simulink model "modelo_f_HIL_ST"  (R2024b)
settings: Solver=ode15s  StartTime=0.0  StopTime=inf  FixedStep=T_s  RelTol=1e-3
InitFcn:
  | clc
  | clear
  | close all
  | clear all
  | clear mex
  | parametros
  | gain_CL
  | calculo_observador_carro
  | calculo_observador_izaje
values from neighbouring files (symbols this model uses):
  b_cx = 1e6    (= 1000000)    [parametros.m]
  b_cy = 1e7    (= 10000000)    [parametros.m]
  b_hb = 1e8    (= 100000000)    [parametros.m]
  b_hd = 8    [parametros.m]
  b_hm = 18    [parametros.m]
  b_t = 90    [parametros.m]
  b_tb = 5e6    (= 5000000)    [parametros.m]
  b_td = 1.8    [parametros.m]
  b_tm = 6    [parametros.m]
  b_tw = 3e3    (= 3000)    [parametros.m]
  b_wu = 150    [parametros.m]
  container_pillars = container_pillars(randperm(19))    [parametros.m]
  escenario = 1    [parametros.m]
  g = 9.80665    [parametros.m]
  H_c = 2.59    [parametros.m]
  H_truck = 1    [parametros.m]
  i_h = 22    [parametros.m]
  i_t = 30    [parametros.m]
  J_hd_hEb = 3800    [parametros.m]
  J_hm_hb = 30    [parametros.m]
  J_td = 1200    [parametros.m]
  J_tm_tb = 7    [parametros.m]
  K_cy = 1.8e9    (= 1800000000)    [parametros.m]
  K_tw = 4.8e5    (= 480000)    [parametros.m]
  k_wu = 2.36e8    (= 236000000)    [parametros.m]
  l_h0 = (Y_t0-y_l0)    (= 38)    [parametros.m]
  l_h_max = Y_t0-y_h_min    (= 65)    [parametros.m]
  l_h_maxE = l_h_max+0.5    (= 65.5)    [parametros.m]
  l_h_min = Y_t0-y_h_max    (= 5)    [parametros.m]
  l_h_minE = l_h_min-0.5    (= 4.5)    [parametros.m]
  M_cmax = 50000    [parametros.m]
  M_cmin = 2000    [parametros.m]
  M_s = 15000    [parametros.m]
  M_t = 30000    [parametros.m]
  r_hd = 0.75    [parametros.m]
  r_td = 0.50    (= 0.5)    [parametros.m]
  T_hbMax = 5e4    (= 50000)    [parametros.m]
  T_hEbMax = 1.1e6    (= 1100000)    [parametros.m]
  T_hmMax = 2e4    (= 20000)    [parametros.m]
  T_s = 0.001    [parametros.m]
  T_s0 = 0.001    [parametros.m]
  T_s1 = 0.020    (= 0.02)    [parametros.m]
  T_s2 = 0.020    (= 0.02)    [parametros.m]
  T_tbMax = 5e3    (= 5000)    [parametros.m]
  T_tmMax = 4e3    (= 4000)    [parametros.m]
  tau_tm = 1e-3    (= 0.001)    [parametros.m]
  theta_hm0 = -l_h0*i_h*2/r_hd    (= -2229.33333333)    [parametros.m]
  theta_tm0 = (x_t0)*i_t/r_td    (= -900)    [parametros.m]
  trucks0 = [0, 0, 0, 0, 0]    [parametros.m]
  v_h_max_load = 1.5    [parametros.m]
  v_h_max_noload = 3    [parametros.m]
  v_lx0 = 0    [parametros.m]
  v_ly0 = 0    [parametros.m]
  v_t0 = 0    [parametros.m]
  v_t_max = 4    [parametros.m]
  W_c = ctrb(A, B_c(:,1))    [CyO_carro.m]    (also in CyO_izaje.m; parametros.m = 2.44)
  w_hm0 = 0    [parametros.m]
  w_hm_rated = v_h_max_load*2*i_h/r_hd    (= 88)    [parametros.m]
  w_tm0 = (v_t0)*i_t/r_td    (= 0)    [parametros.m]
  x_c0_left = -35    [parametros.m]
  x_c0_right = 55    [parametros.m]
  x_containers_left_lim = 1.5    [parametros.m]
  x_containers_right_lim = 48.5    [parametros.m]
  x_l0 = x_t0    (= -15)    [parametros.m]
  x_lidar_offset = 3.0    (= 3)    [parametros.m]
  x_t0 = -15    [parametros.m]
  x_t_max = 50    [parametros.m]
  x_t_maxE = x_t_max+0.5    (= 50.5)    [parametros.m]
  x_t_min = -30    [parametros.m]
  x_t_minE = x_t_min-0.5    (= -30.5)    [parametros.m]
  y_h_min = -20    [parametros.m]
  y_l0 = 7    [parametros.m]
  Y_sb = 5.0    (= 5)    [parametros.m]
  Y_t0 = 45    [parametros.m]
libraries: opcualib x2, dspnetwork x2, dspsigops x1, simulink x1
(part 2 of 3)

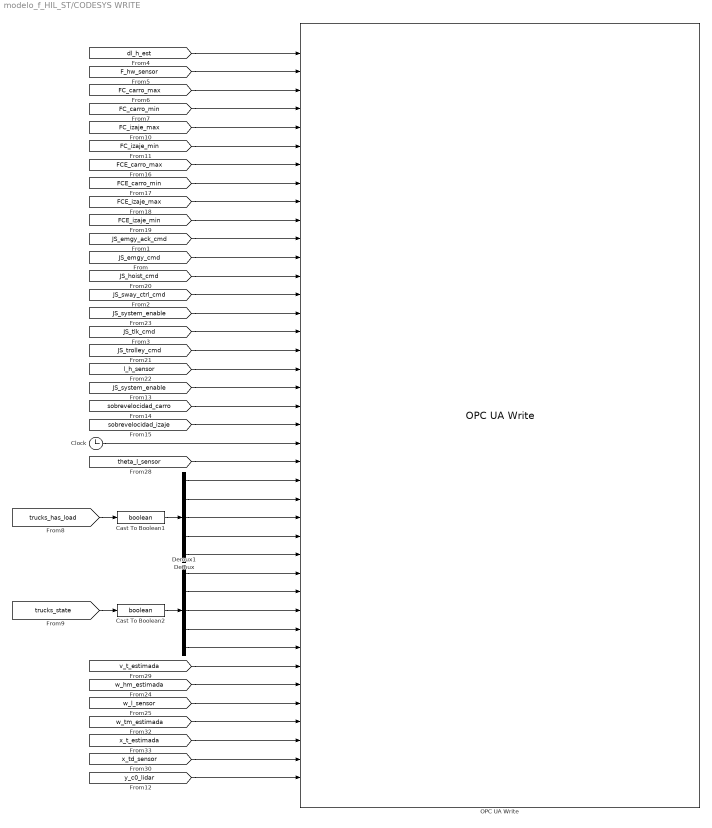
== system modelo_f_HIL_ST/CODESYS WRITE ==
  Cast To Boolean1 : DataTypeConversion  OutDataTypeStr=boolean  SaturateOnIntegerOverflow=off  RndMeth=Floor
  Cast To Boolean2 : DataTypeConversion  OutDataTypeStr=boolean  SaturateOnIntegerOverflow=off  RndMeth=Floor
  Clock : Clock
      settings: Decimation=1/T_s1
  Demux : Demux  Outputs=5
  Demux1 : Demux  Outputs=5
  OPC UA Write : opcualib/OPC UA Write  SelectedServer=OPCUAServer@DESKTOP-IGNACIOMARTINDUCI  ServerList=OPCUAServer@DESKTOP-IGNACIOMARTINDUCI  SampleTime=T_s1  NodeList={ '1', 'dl_h_est', '4', '|var|CODESYS Control Win V3 x64.Application_ST.GVL_VARS.dl_h_est', '0'; '2', 'F_hw_sensor', '4', '|var|CODESYS Control Win V3 x64.Application_ST.GVL_VARS.F_hw_sensor', '0'; '3', 'FC_carro_max', '4', '|var|CODESYS Control Win V3 x64.Application_ST.GVL_VARS.FC_carro_max', '0'; '4', 'FC_carro_min', '4', '|var|CODESYS Control Win V3 x64.Application_ST.GVL_VARS.FC_carro_min', '0'; '5', 'FC_izaje_max', '4', '|var|CODESYS Control Win V3 x64.Application_ST.GVL_VARS.FC_izaje_max', '0'; '6', 'FC_izaje_min', '4', '|var|CODESYS Control Win V3 x64.Application_ST.GVL_VARS.FC_izaje_min', '0'; '7', 'FCE_carro_max', '4', '|var|CODESYS Control Win V3 x64.Application_ST.GVL_VARS.FCE_carro_max', '0'; '8', 'FCE_carro_min', '4', '|var|CODESYS Control Win V3 x64.Application_ST.GVL_VARS.FCE_carro_min', '0'; '9', 'FCE_izaje_max', '4', '|var|CODESYS Control Win V3 x64.Application_ST.GVL_VARS.FCE_izaje_max', '0'; '10', 'FCE_izaje_min', '4', '|var|CODESYS Control Win V3 x64.Application_ST.GVL_VARS.FCE_izaje_min', '0'; '11', 'JS_emgy_ack_cmd', '4', '|var|CODESYS Control Win V3 x64.Application_ST.GVL_VARS.JS_emgy_ack_cmd', '0'; '12', 'JS_emgy_cmd', '4', '|var|CODESYS Control Win V3 x64.Application_ST.GVL_VARS.JS_emgy_cmd', '0'; '13', 'JS_hoist_cmd', '4', '|var|CODESYS Control Win V3 x64.Application_ST.GVL_VARS.JS_hoist_cmd', '0'; '14', 'JS_sway_ctrl_cmd', '4', '|var|CODESYS Control Win V3 x64.Application_ST.GVL_VARS.JS_sway_ctrl_cmd', '0'; '15', 'JS_system_enable', '4', '|var|CODESYS Control Win V3 x64.Application_ST.GVL_VARS.JS_system_enable', '0'; '16', 'JS_tlk_cmd', '4', '|var|CODESYS Control Win V3 x64.Application_ST.GVL_VARS.JS_tlk_cmd', '0'; '17', 'JS_trolley_cmd', '4', '|var|CODESYS Control Win V3 x64.Application_ST.GVL_VARS.JS_trolley_cmd', '0'; '18', 'l_h_sensor', '4', '|var|CODESYS Control Win V3 x64.Application_ST.GVL_VARS.l_h_sensor', '0'; '19', 'P_APN', '4', '|var|CODESYS Control Win V3 x64.Application_ST.GVL_VARS.P_APN', '0'; '20', 'sobrevelocidad_carro', '4', '|var|CODESYS Control Win V3 x64.Application_ST.GVL_VARS.sobrevelocidad_carro', '0'; '21', 'sobrevelocidad_izaje', '4', '|var|CODESYS Control Win V3 x64.Application_ST.GVL_VARS.sobrevelocidad_izaje', '0'; '22', 't', '4', '|var|CODESYS Control Win V3 x64.Application_ST.GVL_VARS.t', '0'; '23', 'theta_l_sensor', '4', '|var|CODESYS Control Win V3 x64.Application_ST.GVL_VARS.theta_l_sensor', '0'; '24', 'THL_1', '4', '|var|CODESYS Control Win V3 x64.Application_ST.GVL_VARS.THL_1', '0'; '25', 'THL_2', '4', '|var|CODESYS Control Win V3 x64.Application_ST.GVL_VARS.THL_2', '0'; '26', 'THL_3', '4', '|var|CODESYS Control Win V3 x64.Application_ST.GVL_VARS.THL_3', '0'; '27', 'THL_4', '4', '|var|CODESYS Control Win V3 x64.Application_ST.GVL_VARS.THL_4', '0'; '28', 'THL_5', '4', '|var|CODESYS Control Win V3 x64.Application_ST.GVL_VARS.THL_5', '0'; '29', 'TS_1', '4', '|var|CODESYS Control Win V3 x64.Application_ST.GVL_VARS.TS_1', '0'; '30', 'TS_2', '4', '|var|CODESYS Control Win V3 x64.Application_ST.GVL_VARS.TS_2', '0'; '31', 'TS_3', '4', '|var|CODESYS Control Win V3 x64.Application_ST.GVL_VARS.TS_3', '0'; '32', 'TS_4', '4', '|var|CODESYS Control Win V3 x64.Application_ST.GVL_VARS.TS_4', '0'; '33', 'TS_5', '4', '|var|CODESYS Control Win V3 x64.Application_ST.GVL_VARS.TS_5', '0'; '34', 'v_t_est', '4', '|var|CODESYS Control Win V3 x64.Application_ST.GVL_VARS.v_t_est', '0'; '35', 'w_hm_estimada', '4', '|var|CODESYS Control Win V3 x64.Application_ST.GVL_VARS.w_hm_estimada', '0'; '36', 'w_l_sensor', '4', '|var|CODESYS Control Win V3 x64.Application_ST.GVL_VARS.w_l_sensor', '0'; '37', 'w_tm_estimada', '4', '|var|CODESYS Control Win V3 x64.Application_ST.GVL_VARS.w_tm_estimada', '0'; '38', 'x_t_est', '4', '|var|CODESYS Control Win V3 x64.Application_ST.GVL_VARS.x_t_est', '0'; '39', 'x_td_sensor', '4', '|var|CODESYS Control Win V3 x64.Application_ST.GVL_VARS.x_td_sensor', '0'; '40', 'y_c0_lidar', '4', '|var|CODESYS Control Win V3 x64.Application_ST.GVL_VARS.y_c0_lidar', '0' }
  wires:
  [dl_h_est] -> OPC UA Write/1
  [F_hw_sensor] -> OPC UA Write/2
  [trucks_has_load] -> Cast To Boolean1/1
  Cast To Boolean1/1 -> Demux/1
  [trucks_state] -> Cast To Boolean2/1
  Cast To Boolean2/1 -> Demux1/1
  [FC_carro_max] -> OPC UA Write/3
  [FC_carro_min] -> OPC UA Write/4
  [FC_izaje_min] -> OPC UA Write/6
  [FCE_carro_min] -> OPC UA Write/8
  [FC_izaje_max] -> OPC UA Write/5
  [FCE_izaje_max] -> OPC UA Write/9
  [FCE_carro_max] -> OPC UA Write/7
  [FCE_izaje_min] -> OPC UA Write/10
  [JS_emgy_ack_cmd] -> OPC UA Write/11
  [JS_emgy_cmd] -> OPC UA Write/12
  [JS_hoist_cmd] -> OPC UA Write/13
  [JS_sway_ctrl_cmd] -> OPC UA Write/14
  [JS_system_enable] -> OPC UA Write/15
  [JS_tlk_cmd] -> OPC UA Write/16
  [JS_trolley_cmd] -> OPC UA Write/17
  [l_h_sensor] -> OPC UA Write/18
  [JS_system_enable] -> OPC UA Write/19
  [sobrevelocidad_carro] -> OPC UA Write/20
  [sobrevelocidad_izaje] -> OPC UA Write/21
  Clock/1 -> OPC UA Write/22
  [theta_l_sensor] -> OPC UA Write/23
  [v_t_estimada] -> OPC UA Write/34
  [w_hm_estimada] -> OPC UA Write/35
  [w_l_sensor] -> OPC UA Write/36
  [w_tm_estimada] -> OPC UA Write/37
  [x_t_estimada] -> OPC UA Write/38
  [x_td_sensor] -> OPC UA Write/39
  [y_c0_lidar] -> OPC UA Write/40
  Demux/1 -> OPC UA Write/24
  Demux/2 -> OPC UA Write/25
  Demux/3 -> OPC UA Write/26
  Demux/4 -> OPC UA Write/27
  Demux/5 -> OPC UA Write/28
  Demux1/1 -> OPC UA Write/29
  Demux1/2 -> OPC UA Write/30
  Demux1/3 -> OPC UA Write/31
  Demux1/4 -> OPC UA Write/32
  Demux1/5 -> OPC UA Write/33

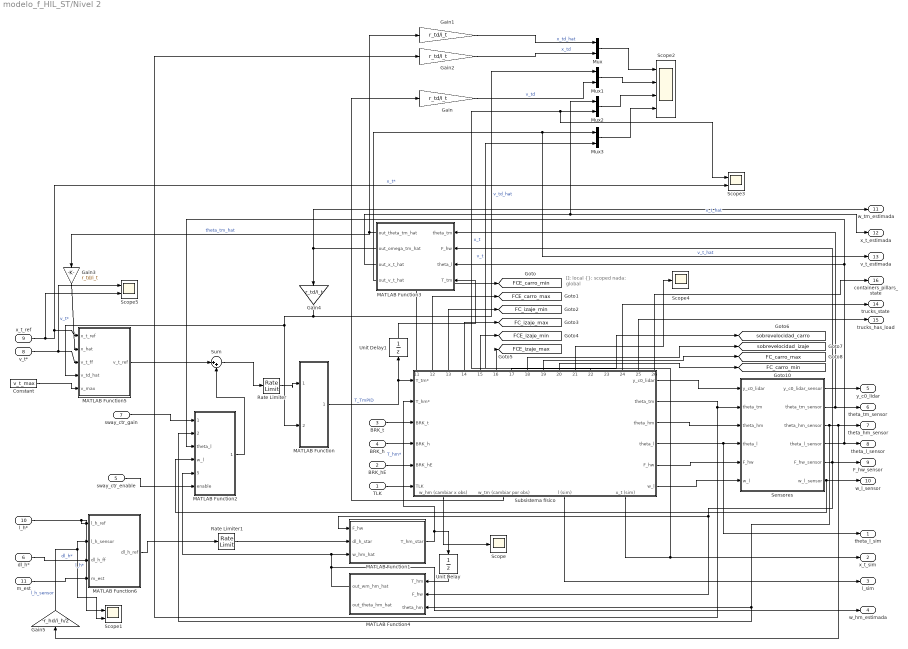
== system modelo_f_HIL_ST/Nivel 2 ==
  note: []: local
      | {}: scoped
      | nada: global
  TLK : Inport
  BRK_hE : Inport  Port=2
  BRK_t : Inport  Port=3
  BRK_h : Inport  Port=4
  sway_ctr_enable : Inport  Port=5
  dl_h* : Inport  Port=6
  sway_ctr_gain : Inport  Port=7
  v_t* : Inport  Port=8
  x_t_ref : Inport  Port=9
  l_h* : Inport  Port=10
  m_est : Inport  Port=11
  Constant : Constant  Value=v_t_max
  Gain{,1..4} (5 alike) : Gain  Gain=r_td/i_t
  Gain5 : Gain  Gain=-r_hd/i_h/2
  MATLAB Function : MATLAB Function  TreatAsAtomicUnit=on  SystemSampleTime=T_s0
  MATLAB Function1 : MATLAB Function  TreatAsAtomicUnit=on  SystemSampleTime=T_s0
  MATLAB Function2 : MATLAB Function  TreatAsAtomicUnit=on  SystemSampleTime=T_s0
  MATLAB Function3 : MATLAB Function  TreatAsAtomicUnit=on  SystemSampleTime=T_s0
  MATLAB Function4 : MATLAB Function  TreatAsAtomicUnit=on  SystemSampleTime=T_s0
  MATLAB Function5 : MATLAB Function  TreatAsAtomicUnit=on
  MATLAB Function6 : MATLAB Function  TreatAsAtomicUnit=on
  Mux{,1..3} (4 alike) : Mux  Inputs=2
  Rate Limiter : RateLimiter  RisingSlewLimit=0.8  FallingSlewLimit=-0.8  SampleTimeMode=inherited  InitialCondition=T_s
  Rate Limiter1 : RateLimiter  RisingSlewLimit=0.75  FallingSlewLimit=-0.75  SampleTimeMode=inherited  InitialCondition=T_s
  Scope : Scope
  Scope1 : Scope  NumInputPorts=2
  Scope2 : Scope  NumInputPorts=4
  Scope3 : Scope  NumInputPorts=2
  Scope4 : Scope
  Scope5 : Scope  NumInputPorts=2
  Sensores : Subsystem
  Subsistema físico : Subsystem
      settings: PortSchema="{\"entries\":[{\"content\":{\"sides\":[{\"content\":{\"connectorIds\":[\"In1\",\"In2\",\"In3\",\"In4\",\"In5\",\"In6\"]},\"type\":\"ConnectorPlacement.EquallySpacedRectSide\",\"uuid\":\"aa1cb789-2051-45a4-8cb8-6dd2078290cc\"},{\"content\":{\"connectorIds\":[\"Out1\",\"Out2\",\"Out3\",\"Out4\",\"Out5\",\"Out6\"],\"side\":\"RIGHT\"},\"type\":\"ConnectorPlacement.EquallySpacedRectSide\",\"uuid\":\"7fe62279-dd3b-46db-ba9e-e4633dcea5c6\"},{\"content\":{\"connectorIds\":[\"Out11\",\"Out12\",\"Out13\",\"Out14\",\"Out15\",\"Out16\",\"Out17\",\"Out18\",\"Out19\",\"Out20\",\"Out21\",\"Out22\",\"Out23\",\"Out24\",\"Out25\",\"Out26\"],\"side\":\"TOP\"},\"type\":\"ConnectorPlacement.EquallySpacedRectSide\",\"uuid\":\"a5663ea7-10d8-47d7-b8ed-8fbfb239b85a\"},{\"content\":{\"connectorIds\":[\"Out7\",\"Out8\",\"Out9\",\"Out10\"],\"side\":\"BOTTOM\"},\"type\":\"ConnectorPlacement.EquallySpacedRectSide\",\"uuid\":\"9ec9131f-7b2f-42d7-8a86-9462c3c282b3\"}]},\"type\":\"ConnectorPlacement.EquallySpacedConnector\",\"uuid\":\"e7df1a56-7803-4e0d-8bf9-081877eb8c08\"}],\"packageUris\":[\"http://schema.mathworks.com/mf0/Connector/R2020b\"],\"version\":\"1.0\"}"
  Sum : Sum  Inputs=|++
  Unit Delay : UnitDelay  SampleTime=T_s  HasFrameUpgradeWarning=on
  Unit Delay1 : UnitDelay  SampleTime=T_s  HasFrameUpgradeWarning=on
  theta_l_sim : Outport
  x_t_sim : Outport  Port=2
  l_sim : Outport  Port=3
  w_hm_estimada : Outport  Port=4
  y_c0_lidar : Outport  Port=5
  theta_tm_sensor : Outport  Port=6
  theta_hm_sensor : Outport  Port=7
  theta_l_sensor : Outport  Port=8
  F_hw_sensor : Outport  Port=9
  w_l_sensor : Outport  Port=10
  w_tm_estimada : Outport  Port=11
  x_t_estimada : Outport  Port=12
  v_t_estimada : Outport  Port=13
  trucks_state : Outport  Port=14
  trucks_has_load : Outport  Port=15
  containers_pillars_state : Outport  Port=16
  tag scope: FCE_carro_max=global, FCE_carro_min=global, FCE_izaje_max=global, FCE_izaje_min=global, FC_carro_max=global, FC_carro_min=global, FC_izaje_max=global, FC_izaje_min=global, sobrevelocidad_carro=global, sobrevelocidad_izaje=global
  wires:
  Sensores/5(F_hw_sensor) -> F_hw_sensor/1, MATLAB Function4/2(F_hw), MATLAB Function1/1(F_hw), MATLAB Function3/2(F_hw)
  Sensores/2(theta_tm_sensor) -> theta_tm_sensor/1, MATLAB Function3/1(theta_tm)
  Subsistema físico/19(FC_carro_max) -> [FC_carro_max]
  Sensores/3(theta_hm_sensor) -> theta_hm_sensor/1, Gain5/1, MATLAB Function4/3(theta_hm), MATLAB Function2/2(theta_hm)
  Sensores/6(w_l_sensor) -> w_l_sensor/1, MATLAB Function2/4(w_l)
  Subsistema físico/15(FCE_izaje_min) -> [FCE_izaje_min]
  Unit Delay/1 -> MATLAB Function4/1(T_hm)
  Subsistema físico/13(FC_izaje_min) -> [FC_izaje_min]
  Subsistema físico/16(FCE_izaje_max) -> [FCE_izaje_max]
  MATLAB Function1/1(T_hm_star) -> Unit Delay/1, Subsistema físico/2(T_hm*)  "T_hm*"
  Subsistema físico/6(w_l) -> Sensores/6(w_l)
  Subsistema físico/17(sobrevelocidad_carro) -> [sobrevelocidad_carro]
  Subsistema físico/3(theta_hm) -> Sensores/3(theta_hm)
  MATLAB Function4/1(out_wm_hm_hat) -> MATLAB Function2/5(w_hm_hat), MATLAB Function1/3(w_hm_hat), w_hm_estimada/1
  dl_h*/1 -> MATLAB Function6/3(dl_h_ff)  "dl_h*"
  Subsistema físico/1(y_c0_lidar) -> Sensores/1(y_c0_lidar)
  Subsistema físico/5(F_hw) -> Sensores/5(F_hw)
  Subsistema físico/2(theta_tm) -> Gain2/1, Sensores/2(theta_tm)
  Subsistema físico/18(sobrevelocidad_izaje) -> [sobrevelocidad_izaje]
  Subsistema físico/11(FCE_carro_min) -> [FCE_carro_min]
  Subsistema físico/4(theta_l) -> theta_l_sim/1, Sensores/4(theta_l)
  Subsistema físico/14(FC_izaje_max) -> [FC_izaje_max]
  Subsistema físico/20(FC_carro_min) -> [FC_carro_min]
  Subsistema físico/12(FCE_carro_max) -> [FCE_carro_max]
  BRK_t/1 -> Subsistema físico/3(BRK_t)
  BRK_h/1 -> Subsistema físico/4(BRK_h)
  BRK_hE/1 -> Subsistema físico/5(BRK_hE)
  TLK/1 -> Subsistema físico/6(TLK)
  Sensores/1(y_c0_lidar_sensor) -> y_c0_lidar/1
  sway_ctr_enable/1 -> MATLAB Function2/6(enable)
  MATLAB Function3/2(out_omega_tm_hat) -> w_tm_estimada/1, Gain4/1
  Gain4/1 -> Mux1/1, MATLAB Function5/4(v_td_hat), MATLAB Function/2(v_td_hat)  "v_td_hat"
  MATLAB Function5/1(v_t_ref) -> Sum/1
  Sensores/4(theta_l_sensor) -> theta_l_sensor/1, MATLAB Function2/3(theta_l), MATLAB Function3/3(theta_l)
  Unit Delay1/1 -> MATLAB Function3/4(T_tm)
  Subsistema físico/10(x_t (sim)) -> Scope3/1, Mux2/2, x_t_sim/1  "x_t"
  Subsistema físico/9(l (sim)) -> l_sim/1
  MATLAB Function3/3(out_x_t_hat) -> x_t_estimada/1, Mux2/1  "x_t_hat"
  Subsistema físico/22(v_t (sim)) -> Mux3/2  "v_t"
  Subsistema físico/8(w_tm (cambiar por obs)) -> Gain/1
  Gain/1 -> Mux1/2  "v_td"
  MATLAB Function3/1(out_theta_tm_hat) -> Gain3/1, Gain1/1  "theta_tm_hat"
  Gain1/1 -> Mux/1  "x_td_hat"
  Gain2/1 -> Mux/2  "x_td"
  MATLAB Function3/4(out_v_t_hat) -> v_t_estimada/1, Mux3/1  "v_t_hat"
  Mux/1 -> Scope2/1
  Mux1/1 -> Scope2/2
  Mux3/1 -> Scope2/4
  Mux2/1 -> Scope2/3
  Subsistema físico/24(trucks_state) -> trucks_state/1
  x_t_ref/1 -> Scope5/2, Scope3/2, MATLAB Function5/1(x_t_ref)  "x_t*"
  sway_ctr_gain/1 -> MATLAB Function2/1(sway_ctr_gain)
  Subsistema físico/25(trucks_has_load) -> trucks_has_load/1
  MATLAB Function/1(T_tm_star) -> Unit Delay1/1, Subsistema físico/1(T_tm*)  "T_TmPID"
  MATLAB Function2/1(v_balanceo) -> Sum/2
  Sum/1 -> Rate Limiter/1
  v_t*/1 -> Scope5/1, MATLAB Function5/3(v_t_ff)  "v_t*"
  Constant/1 -> MATLAB Function5/5(v_max)
  Gain3/1 -> MATLAB Function5/2(x_hat)
  Subsistema físico/7(w_hm (cambiar x obs)) -> Scope/1
  Gain5/1 -> Scope1/2, MATLAB Function6/2(l_h_sensor)  "l_h_sensor"
  l_h*/1 -> Scope1/1, MATLAB Function6/1(l_h_ref)  "l_h*"
  MATLAB Function6/1(dl_h_ref) -> Rate Limiter1/1
  Rate Limiter/1 -> MATLAB Function/1(v_t_star)
  Rate Limiter1/1 -> MATLAB Function1/2(dl_h_star)
  Subsistema físico/26(containers_pillars_state) -> containers_pillars_state/1
  Subsistema físico/21(m_l (sim)) -> Scope4/1
  m_est/1 -> MATLAB Function6/4(m_est)

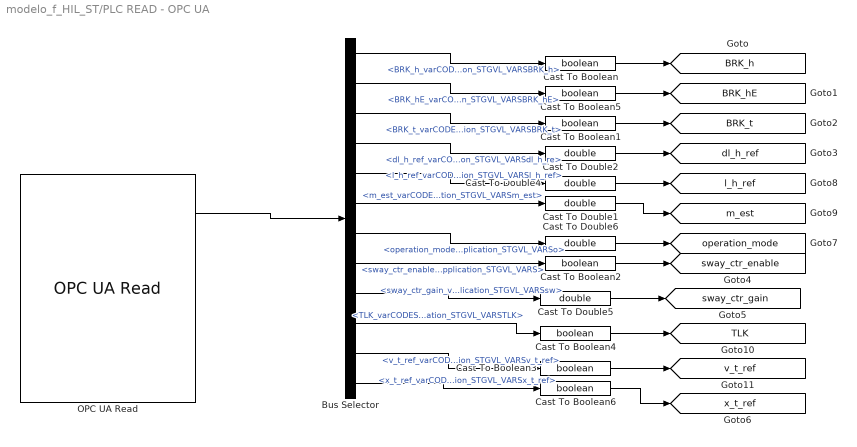
== system modelo_f_HIL_ST/PLC READ - OPC UA ==
  Bus Selector : BusSelector  OutputSignals=BRK_h_varCODESYSControlWinV3X64Application_STGVL_VARSBRK_h,BRK_hE_varCODESYSControlWinV3X64Application_STGVL_VARSBRK_hE,BRK_t_varCODESYSControlWinV3X64Application_STGVL_VARSBRK_t,dl_h_ref_varCODESYSControlWinV3X64Application_STGVL_VARSdl_h_re,l_h_ref_varCODESYSControlWinV3X64Application_STGVL_VARSl_h_ref,m_est_varCODESYSControlWinV3X64Application_STGVL_VARSm_est,operation_mode_varCODESYSControlWinV3X64Application_STGVL_VARSo,sway_ctr_enable_varCODESYSControlWinV3X64Application_STGVL_VARS,sway_ctr_gain_varCODESYSControlWinV3X64Application_STGVL_VARSsw,TLK_varCODESYSControlWinV3X64Application_STGVL_VARSTLK,v_t_ref_varCODESYSControlWinV3X64Application_STGVL_VARSv_t_ref,x_t_ref_varCODESYSControlWinV3X64Application_STGVL_VARSx_t_ref
  Cast To Boolean{,1..6} (7 alike) : DataTypeConversion  OutDataTypeStr=boolean  SaturateOnIntegerOverflow=off  RndMeth=Floor
  Cast To Double{1..2,4..6} (5 alike) : DataTypeConversion  OutDataTypeStr=double  SaturateOnIntegerOverflow=off  RndMeth=Floor
  OPC UA Read : opcualib/OPC UA Read  SelectedServer=OPCUAServer@DESKTOP-IGNACIOMARTINDUCI  ServerList=OPCUAServer@DESKTOP-IGNACIOMARTINDUCI  NodeList={ '1', 'BRK_h', '4', '|var|CODESYS Control Win V3 x64.Application_ST.GVL_VARS.BRK_h', '0'; '2', 'BRK_hE', '4', '|var|CODESYS Control Win V3 x64.Application_ST.GVL_VARS.BRK_hE', '0'; '3', 'BRK_t', '4', '|var|CODESYS Control Win V3 x64.Application_ST.GVL_VARS.BRK_t', '0'; '4', 'dl_h_ref', '4', '|var|CODESYS Control Win V3 x64.Application_ST.GVL_VARS.dl_h_ref', '0'; '5', 'l_h_ref', '4', '|var|CODESYS Control Win V3 x64.Application_ST.GVL_VARS.l_h_ref', '0'; '6', 'm_est', '4', '|var|CODESYS Control Win V3 x64.Application_ST.GVL_VARS.m_est', '0'; '7', 'operation_mode', '4', '|var|CODESYS Control Win V3 x64.Application_ST.GVL_VARS.operation_mode', '0'; '8', 'sway_ctr_enable', '4', '|var|CODESYS Control Win V3 x64.Application_ST.GVL_VARS.sway_ctr_enable', '0'; '9', 'sway_ctr_gain', '4', '|var|CODESYS Control Win V3 x64.Application_ST.GVL_VARS.sway_ctr_gain', '0'; '10', 'TLK', '4', '|var|CODESYS Control Win V3 x64.Application_ST.GVL_VARS.TLK', '0'; '11', 'v_t_ref', '4', '|var|CODESYS Control Win V3 x64.Application_ST.GVL_VARS.v_t_ref', '0'; '12', 'x_t_ref', '4', '|var|CODESYS Control Win V3 x64.Application_ST.GVL_VARS.x_t_ref', '0' }  ShowQualityPort=on  ShowTimestampPort=on  ShowTimestampPortAs=Seconds since start  SampleTime=T_s1
  tag scope: BRK_h=global, BRK_hE=global, BRK_t=global, TLK=global, dl_h_ref=global, l_h_ref=global, m_est=global, operation_mode=global, sway_ctr_enable=global, sway_ctr_gain=global, v_t_ref=global, x_t_ref=global
  wires:
  Bus Selector/1 -> Cast To Boolean/1  "<BRK_h_varCODESYSControlWinV3X64Application_STGVL_VARSBRK_h>"
  Bus Selector/3 -> Cast To Boolean1/1  "<BRK_t_varCODESYSControlWinV3X64Application_STGVL_VARSBRK_t>"
  Bus Selector/9 -> Cast To Double5/1  "<sway_ctr_gain_varCODESYSControlWinV3X64Application_STGVL_VARSsw>"
  Bus Selector/6 -> Cast To Double1/1  "<m_est_varCODESYSControlWinV3X64Application_STGVL_VARSm_est>"
  Bus Selector/2 -> Cast To Boolean5/1  "<BRK_hE_varCODESYSControlWinV3X64Application_STGVL_VARSBRK_hE>"
  Bus Selector/4 -> Cast To Double2/1  "<dl_h_ref_varCODESYSControlWinV3X64Application_STGVL_VARSdl_h_re>"
  Bus Selector/5 -> Cast To Double4/1  "<l_h_ref_varCODESYSControlWinV3X64Application_STGVL_VARSl_h_ref>"
  Bus Selector/10 -> Cast To Boolean4/1  "<TLK_varCODESYSControlWinV3X64Application_STGVL_VARSTLK>"
  Cast To Boolean/1 -> [BRK_h]
  Cast To Boolean5/1 -> [BRK_hE]
  Cast To Boolean1/1 -> [BRK_t]
  Cast To Double2/1 -> [dl_h_ref]
  Cast To Double5/1 -> [sway_ctr_gain]
  Cast To Double4/1 -> [l_h_ref]
  Cast To Double1/1 -> [m_est]
  Cast To Boolean4/1 -> [TLK]
  Cast To Double6/1 -> [operation_mode]
  Bus Selector/7 -> Cast To Double6/1  "<operation_mode_varCODESYSControlWinV3X64Application_STGVL_VARSo>"
  Bus Selector/8 -> Cast To Boolean2/1  "<sway_ctr_enable_varCODESYSControlWinV3X64Application_STGVL_VARS>"
  Cast To Boolean2/1 -> [sway_ctr_enable]
  OPC UA Read/1 -> Bus Selector/1
  Cast To Boolean3/1 -> [v_t_ref]
  Bus Selector/11 -> Cast To Boolean3/1  "<v_t_ref_varCODESYSControlWinV3X64Application_STGVL_VARSv_t_ref>"
  Bus Selector/12 -> Cast To Boolean6/1  "<x_t_ref_varCODESYSControlWinV3X64Application_STGVL_VARSx_t_ref>"
  Cast To Boolean6/1 -> [x_t_ref]

== system modelo_f_HIL_ST/UDP: Controller reader ==
  Cast To Boolean{,2..5} (5 alike) : DataTypeConversion  OutDataTypeStr=boolean  SaturateOnIntegerOverflow=off  RndMeth=Floor
  MATLAB Function : MATLAB Function  TreatAsAtomicUnit=on
  UDP Receive1 : dspnetwork/UDP Receive  localURL='0.0.0.0'  localPort=5005  remoteURL='0.0.0.0'  remotePort=-1  recvBufferSize=14  dims=255  signalDatatype=uint8  isComplex=off  isVarSize=on  showBlockingTime=off  blockingTime=0  sampletime=1  blockPlatform=[]
      settings: LibrarySourceBlock=dspsrcs4/UDP Receive
  tag scope: JS_emgy_ack_cmd=global, JS_emgy_cmd=global, JS_hoist_cmd=global, JS_sway_ctrl_cmd=global, JS_system_enable=global, JS_tlk_cmd=global, JS_trolley_cmd=global
  wires:
  UDP Receive1/1 -> MATLAB Function/1(data)
  MATLAB Function/1(trolley_cmd) -> [JS_trolley_cmd]  "trolley_cmd"
  MATLAB Function/2(hoist_cmd) -> [JS_hoist_cmd]  "hoist_cmd"
  MATLAB Function/3(system_on) -> Cast To Boolean/1  "system_on"
  MATLAB Function/4(twistlock) -> Cast To Boolean2/1  "twistlock"
  MATLAB Function/5(sway_ctrl) -> Cast To Boolean3/1  "sway_ctrl"
  MATLAB Function/6(emergency) -> Cast To Boolean4/1  "emergency"
  MATLAB Function/7(emgy_ack) -> Cast To Boolean5/1  "emgy ack"
  Cast To Boolean/1 -> [JS_system_enable]
  Cast To Boolean2/1 -> [JS_tlk_cmd]
  Cast To Boolean4/1 -> [JS_emgy_cmd]
  Cast To Boolean5/1 -> [JS_emgy_ack_cmd]
  Cast To Boolean3/1 -> [JS_sway_ctrl_cmd]

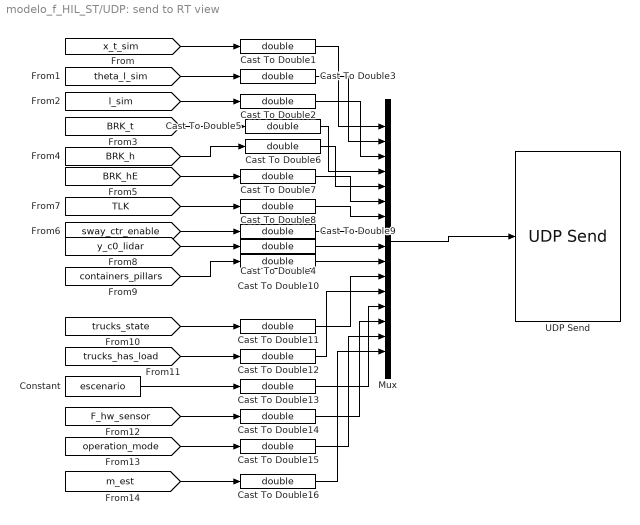
== system modelo_f_HIL_ST/UDP: send to RT view ==
  Cast To Double{1..16} (16 alike) : DataTypeConversion  OutDataTypeStr=double  SaturateOnIntegerOverflow=off  RndMeth=Floor
  Constant : Constant  Value=escenario
  Mux : Mux  Inputs=16
  UDP Send : dspnetwork/UDP Send  remoteURL='127.0.0.1'  remotePort=5010  localURL='0.0.0.0'  localPortSource=Automatically determine  localPort=-1  sendBufferSize=8192  sampletime=-1  blockPlatform=[]  separateLengthPort=0
      settings: LibrarySourceBlock=dspsnks4/UDP Send
  wires:
  [x_t_sim] -> Cast To Double1/1
  [theta_l_sim] -> Cast To Double3/1
  Mux/1 -> UDP Send/1
  [l_sim] -> Cast To Double2/1
  [BRK_t] -> Cast To Double5/1
  [BRK_h] -> Cast To Double6/1
  [BRK_hE] -> Cast To Double7/1
  [sway_ctr_enable] -> Cast To Double9/1
  [TLK] -> Cast To Double8/1
  Cast To Double1/1 -> Mux/1
  Cast To Double3/1 -> Mux/2
  Cast To Double2/1 -> Mux/3
  Cast To Double5/1 -> Mux/4
  Cast To Double6/1 -> Mux/5
  Cast To Double7/1 -> Mux/6
  Cast To Double8/1 -> Mux/7
  Cast To Double9/1 -> Mux/8
  [y_c0_lidar] -> Cast To Double4/1
  Cast To Double4/1 -> Mux/9
  [containers_pillars] -> Cast To Double10/1
  Cast To Double10/1 -> Mux/10
  [trucks_state] -> Cast To Double11/1
  Cast To Double11/1 -> Mux/11
  [trucks_has_load] -> Cast To Double12/1
  Cast To Double12/1 -> Mux/12
  Cast To Double13/1 -> Mux/13
  Constant/1 -> Cast To Double13/1
  Cast To Double14/1 -> Mux/14
  [F_hw_sensor] -> Cast To Double14/1
  [operation_mode] -> Cast To Double15/1
  Cast To Double15/1 -> Mux/15
  [m_est] -> Cast To Double16/1
  Cast To Double16/1 -> Mux/16

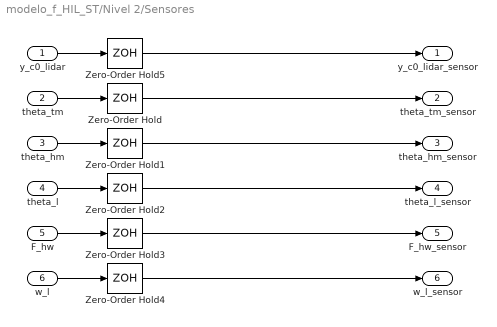
== system modelo_f_HIL_ST/Nivel 2/Sensores ==
  y_c0_lidar : Inport
  theta_tm : Inport  Port=2
  theta_hm : Inport  Port=3
  theta_l : Inport  Port=4
  F_hw : Inport  Port=5
  w_l : Inport  Port=6
  Zero-Order Hold{,2..5} (5 alike) : ZeroOrderHold  SampleTime=T_s
  Zero-Order Hold1 : ZeroOrderHold  SampleTime=T_s2
  y_c0_lidar_sensor : Outport
  theta_tm_sensor : Outport  Port=2
  theta_hm_sensor : Outport  Port=3
  theta_l_sensor : Outport  Port=4
  F_hw_sensor : Outport  Port=5
  w_l_sensor : Outport  Port=6
  wires:
  theta_tm/1 -> Zero-Order Hold/1
  Zero-Order Hold/1 -> theta_tm_sensor/1
  Zero-Order Hold1/1 -> theta_hm_sensor/1
  theta_hm/1 -> Zero-Order Hold1/1
  w_l/1 -> Zero-Order Hold4/1
  F_hw/1 -> Zero-Order Hold3/1
  theta_l/1 -> Zero-Order Hold2/1
  Zero-Order Hold2/1 -> theta_l_sensor/1
  Zero-Order Hold3/1 -> F_hw_sensor/1
  Zero-Order Hold4/1 -> w_l_sensor/1
  Zero-Order Hold5/1 -> y_c0_lidar_sensor/1
  y_c0_lidar/1 -> Zero-Order Hold5/1

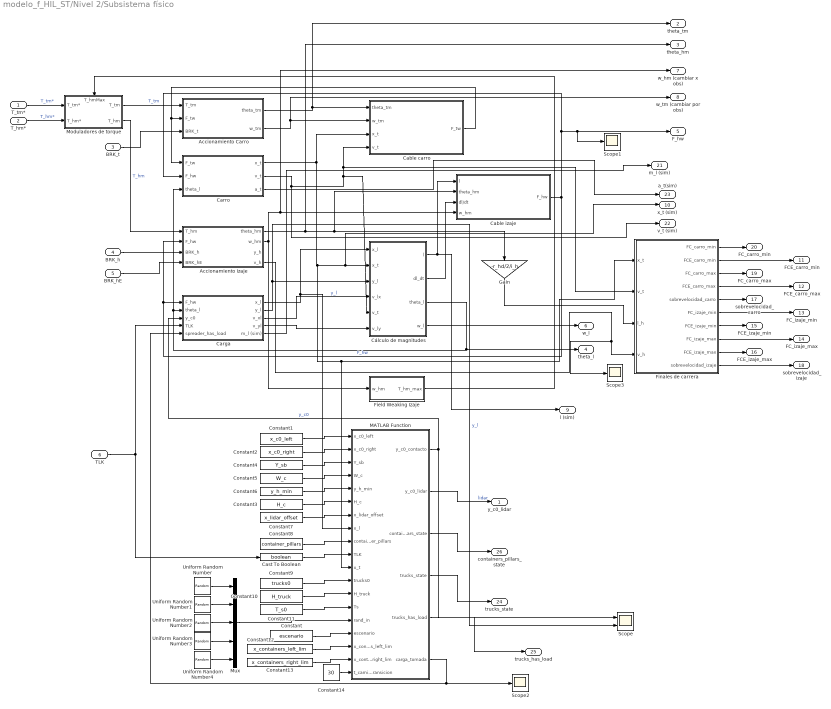
== system modelo_f_HIL_ST/Nivel 2/Subsistema físico ==
  T_tm* : Inport
  T_hm* : Inport  Port=2
  BRK_t : Inport  Port=3
  BRK_h : Inport  Port=4
  BRK_hE : Inport  Port=5
  TLK : Inport  Port=6
  Accionamiento Carro : Subsystem
  Accionamiento Izaje : Subsystem
  Cable carro : Subsystem
  Cable izaje : Subsystem
  Carga : Subsystem
  Carro : Subsystem
  Cast To Boolean : DataTypeConversion  OutDataTypeStr=boolean  SaturateOnIntegerOverflow=off  RndMeth=Floor
  Constant : Constant  Value=escenario
  Constant1 : Constant  Value=x_c0_left
  Constant10 : Constant  Value=H_truck
  Constant11 : Constant  Value=T_s0
  Constant12 : Constant  Value=x_containers_left_lim
  Constant13 : Constant  Value=x_containers_right_lim
  Constant14 : Constant  Value=30
  Constant2 : Constant  Value=x_c0_right
  Constant3 : Constant  Value=H_c
  Constant4 : Constant  Value=Y_sb
  Constant5 : Constant  Value=W_c
  Constant6 : Constant  Value=y_h_min
  Constant7 : Constant  Value=x_lidar_offset
  Constant8 : Constant  Value=container_pillars
  Constant9 : Constant  Value=trucks0
  Cálculo de magnitudes : Subsystem
  Field Weaking Izaje : Subsystem
  Finales de carrera : Subsystem
  Gain : Gain  Gain=-r_hd/2/i_h
  MATLAB Function : MATLAB Function  TreatAsAtomicUnit=on  SystemSampleTime=T_s
  Moduladores de torque : Subsystem
      settings: PortSchema="{\"entries\":[{\"content\":{\"sides\":[{\"content\":{\"connectorIds\":[\"In1\",\"In2\"]},\"type\":\"ConnectorPlacement.EquallySpacedRectSide\",\"uuid\":\"c66d3892-523c-433a-8dde-517eb495bac1\"},{\"content\":{\"connectorIds\":[\"Out1\",\"Out2\"],\"side\":\"RIGHT\"},\"type\":\"ConnectorPlacement.EquallySpacedRectSide\",\"uuid\":\"bbb0a9b0-6ff9-4fa8-ace8-11da5b7abadd\"},{\"content\":{\"connectorIds\":[\"In3\"],\"side\":\"TOP\"},\"type\":\"ConnectorPlacement.EquallySpacedRectSide\",\"uuid\":\"35baaaad-8e6c-401a-84f7-749de5492b29\"}]},\"type\":\"ConnectorPlacement.EquallySpacedConnector\",\"uuid\":\"d8d05b6c-004b-40f1-854a-ea077232777a\"}],\"packageUris\":[\"http://schema.mathworks.com/mf0/Connector/R2020b\"],\"version\":\"1.0\"}"
  Mux : Mux  Inputs=5
  Scope : Scope  NumInputPorts=2
  Scope1 : Scope
  Scope2 : Scope
  Scope3 : Scope
  Uniform Random Number : UniformRandomNumber  Minimum=0  Seed=12415  SampleTime=T_s0
  Uniform Random Number1 : UniformRandomNumber  Minimum=0  Seed=3123  SampleTime=T_s0
  Uniform Random Number2 : UniformRandomNumber  Minimum=0  Seed=123124  SampleTime=T_s0
  Uniform Random Number3 : UniformRandomNumber  Minimum=0  Seed=28682  SampleTime=T_s0
  Uniform Random Number4 : UniformRandomNumber  Minimum=0  Seed=999  SampleTime=T_s0
  y_c0_lidar : Outport
  theta_tm : Outport  Port=2
  theta_hm : Outport  Port=3
  theta_l : Outport  Port=4
  F_hw : Outport  Port=5
  w_l : Outport  Port=6
  w_hm (cambiar x obs) : Outport  Port=7
  w_tm (cambiar por obs) : Outport  Port=8
  l (sim) : Outport  Port=9
  x_t (sim) : Outport  Port=10
  FCE_carro_min : Outport  Port=11
  FCE_carro_max : Outport  Port=12
  FC_izaje_min : Outport  Port=13
  FC_izaje_max : Outport  Port=14
  FCE_izaje_min : Outport  Port=15
  FCE_izaje_max : Outport  Port=16
  sobrevelocidad_carro : Outport  Port=17
  sobrevelocidad_izaje : Outport  Port=18
  FC_carro_max : Outport  Port=19
  FC_carro_min : Outport  Port=20
  m_l (sim) : Outport  Port=21
  v_t (sim) : Outport  Port=22
  a_t(sim) : Outport  Port=23
  trucks_state : Outport  Port=24
  trucks_has_load : Outport  Port=25
  containers_pillars_state : Outport  Port=26
  wires:
  T_tm*/1 -> Moduladores de torque/1(T_tm*)  "T_tm*"
  Accionamiento Carro/1(theta_tm) -> theta_tm/1, Cable carro/1(theta_tm)
  Accionamiento Carro/2(w_tm) -> w_tm (cambiar por obs)/1, Cable carro/2(w_tm)
  Carro/1(x_t) -> Finales de carrera/1(x_t), MATLAB Function/11(x_t), x_t (sim)/1, Cálculo de magnitudes/2(x_t), Cable carro/3(x_t)
  Carro/2(v_t) -> v_t (sim)/1, Cálculo de magnitudes/5(v_t), Cable carro/4(v_t), Finales de carrera/2(v_t)
  Cable carro/1(F_tw) -> Carro/1(F_tw), Accionamiento Carro/2(F_tw)
  Carga/1(x_l) -> MATLAB Function/8(x_l), Cálculo de magnitudes/1(x_l)
  Carga/2(y_l) -> Scope/2, Cálculo de magnitudes/3(y_l)  "y_l"
  Carga/3(v_xl) -> Cálculo de magnitudes/4(v_lx)  "y_l"
  Carga/4(v_yl) -> Cálculo de magnitudes/6(v_ly)
  Cálculo de magnitudes/1(l) -> l (sim)/1, Cable izaje/1(l)
  Accionamiento Izaje/1(theta_hm) -> Gain/1, Cable izaje/2(theta_hm), theta_hm/1
  Cálculo de magnitudes/2(dl_dt) -> Cable izaje/3(dl/dt)
  T_hm*/1 -> Moduladores de torque/2(T_hm*)  "T_hm*"
  Accionamiento Izaje/2(w_hm) -> w_hm (cambiar x obs)/1, Cable izaje/4(w_hm), Field Weaking Izaje/1(w_hm)
  BRK_t/1 -> Accionamiento Carro/3(BRK_t)
  BRK_h/1 -> Accionamiento Izaje/3(BRK_h)
  BRK_hE/1 -> Accionamiento Izaje/4(BRK_hE)
  Accionamiento Izaje/4(v_h) -> Finales de carrera/4(v_h), Scope3/1
  Cálculo de magnitudes/4(w_l) -> w_l/1
  Moduladores de torque/1(T_tm) -> Accionamiento Carro/1(T_tm)  "T_tm"
  Field Weaking Izaje/1(T_hm_max) -> Moduladores de torque/3(T_hmMax)
  Moduladores de torque/2(T_hm) -> Accionamiento Izaje/1(T_hm)  "T_hm"
  Finales de carrera/1(FC_carro_min) -> FC_carro_min/1
  Finales de carrera/2(FCE_carro_min) -> FCE_carro_min/1
  Finales de carrera/3(FC_carro_max) -> FC_carro_max/1
  Finales de carrera/4(FCE_carro_max) -> FCE_carro_max/1
  Finales de carrera/5(sobrevelocidad_carro) -> sobrevelocidad_carro/1
  Finales de carrera/7(FCE_izaje_min) -> FCE_izaje_min/1
  Finales de carrera/6(FC_izaje_min) -> FC_izaje_min/1
  Finales de carrera/8(FC_izaje_max) -> FC_izaje_max/1
  Finales de carrera/9(FCE_izaje_max) -> FCE_izaje_max/1
  Finales de carrera/10(sobrevelocidad_izaje) -> sobrevelocidad_izaje/1
  Constant1/1 -> MATLAB Function/1(x_c0_left)
  Constant2/1 -> MATLAB Function/2(x_c0_right)
  Constant3/1 -> MATLAB Function/6(H_c)
  Constant4/1 -> MATLAB Function/3(Y_sb)
  Constant5/1 -> MATLAB Function/4(W_c)
  Constant6/1 -> MATLAB Function/5(y_h_min)
  MATLAB Function/1(y_c0_contacto) -> Scope/1, Carga/3(y_c0)  "y_c0"
  Constant7/1 -> MATLAB Function/7(x_lidar_offset)
  Gain/1 -> Finales de carrera/3(l_h)
  Carga/5(m_l (sim)) -> m_l (sim)/1
  Cálculo de magnitudes/3(theta_l) -> Carro/3(theta_l), Carga/2(theta_l), theta_l/1
  Carro/3(a_t) -> a_t(sim)/1
  MATLAB Function/2(y_c0_lidar) -> y_c0_lidar/1  "lidar"
  Constant8/1 -> MATLAB Function/9(container_pillars)
  MATLAB Function/4(trucks_state) -> trucks_state/1
  Constant9/1 -> MATLAB Function/12(trucks0)
  Constant10/1 -> MATLAB Function/13(H_truck)
  Constant11/1 -> MATLAB Function/14(Ts)
  Uniform Random Number1/1 -> Mux/2
  Uniform Random Number/1 -> Mux/1
  Uniform Random Number2/1 -> Mux/3
  Uniform Random Number3/1 -> Mux/4
  Uniform Random Number4/1 -> Mux/5
  Constant/1 -> MATLAB Function/16(escenario)
  MATLAB Function/5(trucks_has_load) -> trucks_has_load/1
  Constant12/1 -> MATLAB Function/17(x_containers_left_lim)
  Constant13/1 -> MATLAB Function/18(x_containers_right_lim)
  MATLAB Function/3(containers_pillars_state) -> containers_pillars_state/1
  TLK/1 -> Cast To Boolean/1, Carga/4(TLK)
  Cast To Boolean/1 -> MATLAB Function/10(TLK)
  Mux/1 -> MATLAB Function/15(rand_in)
  Cable izaje/1(F_hw) -> Carro/2(F_hw), Scope1/1, F_hw/1, Accionamiento Izaje/2(F_hw), Carga/1(F_hw)  "F_hw"
  MATLAB Function/6(carga_tomada) -> Scope2/1, Carga/5(spreader_has_load)
  Constant14/1 -> MATLAB Function/19(t_camion_transicion)

== system modelo_f_HIL_ST/Nivel 2/Subsistema físico/Accionamiento Carro ==
  T_tm : Inport
  F_tw : Inport  Port=2
  BRK_t : Inport  Port=3
  Gain : Gain  Gain=1/(J_tm_tb+J_td/i_t^2)
  Gain1 : Gain  Gain=r_td/i_t
  Gain2 : Gain  Gain=(b_tm+b_td/i_t^2)
  Integrator : Integrator  InitialCondition=w_tm0
  Integrator1 : Integrator  InitialCondition=theta_tm0
  Subsystem : Subsystem
  Sum : Sum  Inputs=+-+-
  theta_tm : Outport
  w_tm : Outport  Port=2
  wires:
  Integrator1/1 -> theta_tm/1
  Integrator/1 -> w_tm/1, Gain2/1, Subsystem/2(w_tm), Integrator1/1  "w_tm"
  Gain/1 -> Integrator/1
  Sum/1 -> Gain/1
  T_tm/1 -> Sum/1
  F_tw/1 -> Gain1/1
  Gain1/1 -> Sum/2
  Subsystem/1(T_tb) -> Sum/3
  Gain2/1 -> Sum/4
  BRK_t/1 -> Subsystem/1(BRK_t)

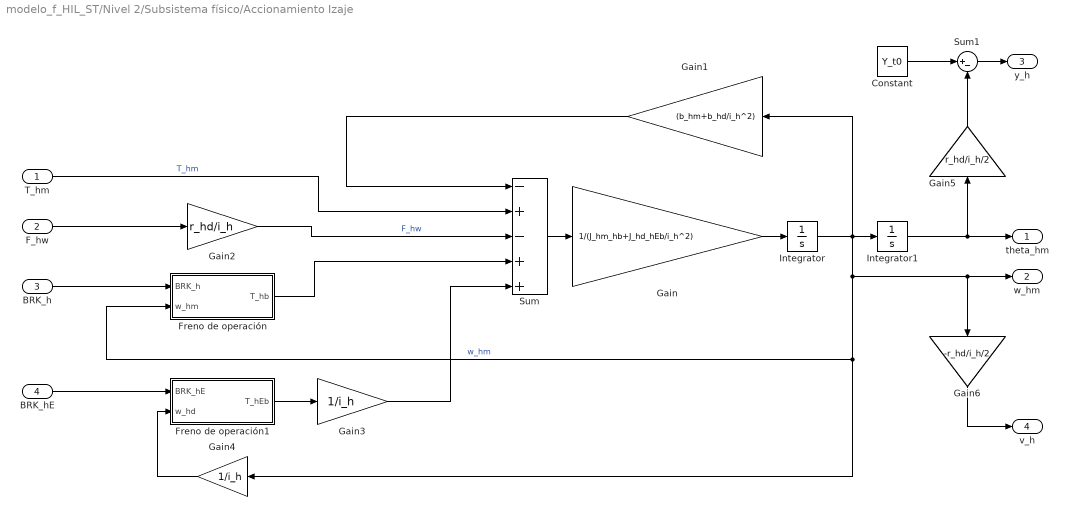
== system modelo_f_HIL_ST/Nivel 2/Subsistema físico/Accionamiento Izaje ==
  T_hm : Inport
  F_hw : Inport  Port=2
  BRK_h : Inport  Port=3
  BRK_hE : Inport  Port=4
  Constant : Constant  Value=Y_t0
  Freno de operación : Subsystem
  Freno de operación1 : Subsystem
  Gain : Gain  Gain=1/(J_hm_hb+J_hd_hEb/i_h^2)
  Gain1 : Gain  Gain=(b_hm+b_hd/i_h^2)
  Gain2 : Gain  Gain=r_hd/i_h
  Gain3 : Gain  Gain=1/i_h
  Gain4 : Gain  Gain=1/i_h
  Gain5 : Gain  Gain=r_hd/i_h/2
  Gain6 : Gain  Gain=-r_hd/i_h/2
  Integrator : Integrator  InitialCondition=w_hm0
  Integrator1 : Integrator  InitialCondition=theta_hm0
  Sum : Sum  Inputs=-+-++
  Sum1 : Sum  Inputs=|+-
  theta_hm : Outport
  w_hm : Outport  Port=2
  y_h : Outport  Port=3
  v_h : Outport  Port=4
  wires:
  Integrator1/1 -> Gain5/1, theta_hm/1
  Integrator/1 -> Integrator1/1, Gain6/1, w_hm/1, Gain4/1, Freno de operación/2(w_hm), Gain1/1  "w_hm"
  Gain/1 -> Integrator/1
  Sum/1 -> Gain/1
  Gain1/1 -> Sum/1
  F_hw/1 -> Gain2/1
  Gain2/1 -> Sum/3  "F_hw"
  T_hm/1 -> Sum/2  "T_hm"
  Freno de operación/1(T_hb) -> Sum/4
  BRK_h/1 -> Freno de operación/1(BRK_h)
  Freno de operación1/1(T_hEb) -> Gain3/1
  Gain3/1 -> Sum/5
  BRK_hE/1 -> Freno de operación1/1(BRK_hE)
  Gain4/1 -> Freno de operación1/2(w_hd)
  Sum1/1 -> y_h/1
  Gain5/1 -> Sum1/2
  Constant/1 -> Sum1/1
  Gain6/1 -> v_h/1

== system modelo_f_HIL_ST/Nivel 2/Subsistema físico/Cable carro ==
  theta_tm : Inport
  w_tm : Inport  Port=2
  x_t : Inport  Port=3
  v_t : Inport  Port=4
  Gain : Gain  Gain=b_tw
  Gain1 : Gain  Gain=K_tw
  Gain2 : Gain  Gain=r_td/i_t
  Gain3 : Gain  Gain=r_td/i_t
  Sum : Sum  Inputs=|+-
  Sum1 : Sum  Inputs=|+-
  Sum2 : Sum  Inputs=|++
  F_tw : Outport
  wires:
  Sum/1 -> Gain1/1
  theta_tm/1 -> Gain3/1
  x_t/1 -> Sum/2
  Sum1/1 -> Gain/1
  w_tm/1 -> Gain2/1
  v_t/1 -> Sum1/2
  Gain/1 -> Sum2/2
  Gain1/1 -> Sum2/1
  Sum2/1 -> F_tw/1
  Gain2/1 -> Sum1/1  "v_td"
  Gain3/1 -> Sum/1  "x_td"

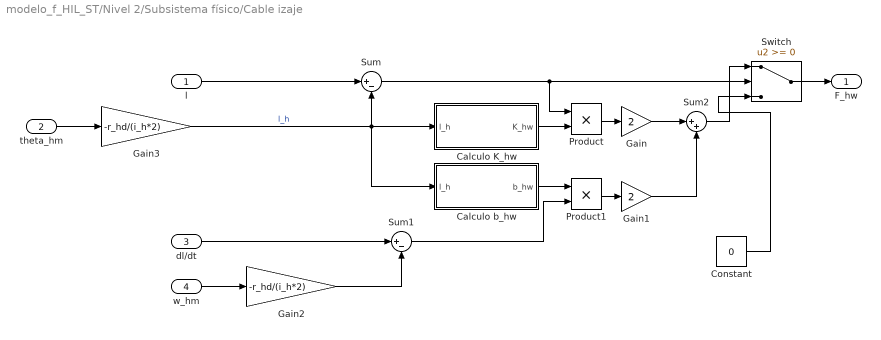
== system modelo_f_HIL_ST/Nivel 2/Subsistema físico/Cable izaje ==
  l : Inport
  theta_hm : Inport  Port=2
  dl/dt : Inport  Port=3
  w_hm : Inport  Port=4
  Calculo K_hw : Subsystem
  Calculo b_hw : Subsystem
  Constant : Constant  Value=0
  Gain : Gain  Gain=2
  Gain1 : Gain  Gain=2
  Gain2 : Gain  Gain=-r_hd/(i_h*2)
  Gain3 : Gain  Gain=-r_hd/(i_h*2)
  Product : Product
  Product1 : Product
  Sum : Sum  Inputs=|+-
  Sum1 : Sum  Inputs=|+-
  Sum2 : Sum  Inputs=|++
  Switch : Switch  SaturateOnIntegerOverflow=off  InputSameDT=off
  F_hw : Outport
  wires:
  l/1 -> Sum/1
  theta_hm/1 -> Gain3/1
  Sum/1 -> Product/1, Switch/2
  Calculo K_hw/1(K_hw) -> Product/2
  Product/1 -> Gain/1
  w_hm/1 -> Gain2/1
  Product1/1 -> Gain1/1
  Calculo b_hw/1(b_hw) -> Product1/1
  Gain1/1 -> Sum2/2
  Gain/1 -> Sum2/1
  Sum2/1 -> Switch/1
  Switch/1 -> F_hw/1
  dl/dt/1 -> Sum1/1
  Constant/1 -> Switch/3
  Gain2/1 -> Sum1/2
  Gain3/1 -> Calculo b_hw/1(l_h), Calculo K_hw/1(l_h), Sum/2  "l_h"
  Sum1/1 -> Product1/2

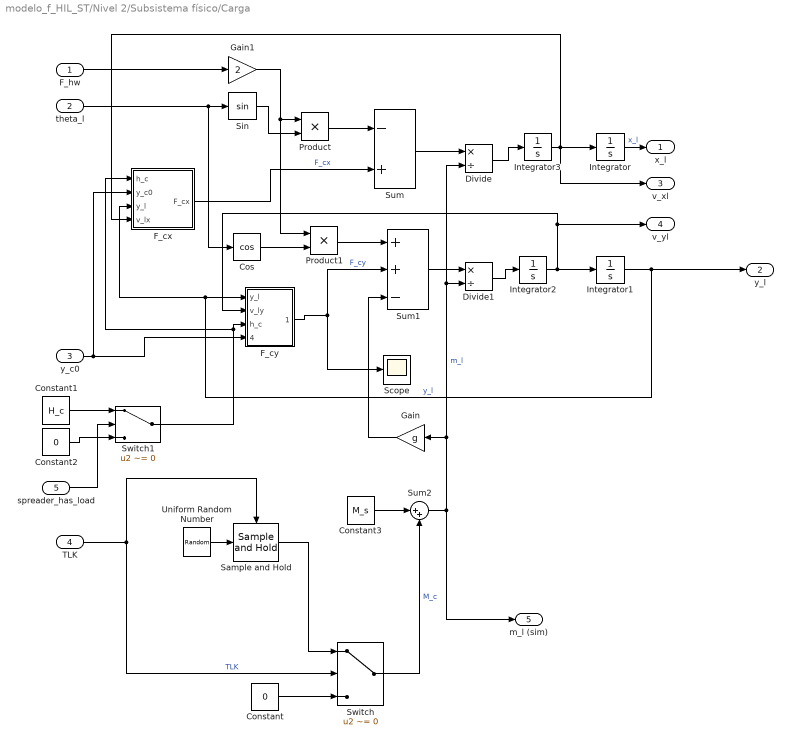
== system modelo_f_HIL_ST/Nivel 2/Subsistema físico/Carga ==
  F_hw : Inport
  theta_l : Inport  Port=2
  y_c0 : Inport  Port=3
  TLK : Inport  Port=4
  spreader_has_load : Inport  Port=5
  Constant : Constant  Value=0
  Constant1 : Constant  Value=H_c
  Constant2 : Constant  Value=0
  Constant3 : Constant  Value=M_s
  Cos : Trigonometry  Operator=cos
  Divide : Product  Inputs=*/
  Divide1 : Product  Inputs=*/
  F_cx : Subsystem
  F_cy : Subsystem
  Gain : Gain  Gain=g
  Gain1 : Gain  Gain=2
  Integrator : Integrator  InitialCondition=x_l0
  Integrator1 : Integrator  InitialCondition=y_l0
  Integrator2 : Integrator  InitialCondition=v_ly0
  Integrator3 : Integrator  InitialCondition=v_lx0
  Product : Product
  Product1 : Product
  Sample and Hold : dspsigops/Sample and Hold  trig=Rising edge  initCond=0  latchinput=off
  Scope : Scope
  Sin : Trigonometry
  Sum : Sum  Inputs=-+
  Sum1 : Sum  Inputs=++-
  Sum2 : Sum  Inputs=|++
  Switch : Switch  Criteria=u2 ~= 0  SaturateOnIntegerOverflow=off  InputSameDT=off
  Switch1 : Switch  Criteria=u2 ~= 0  SaturateOnIntegerOverflow=off  InputSameDT=off
  Uniform Random Number : UniformRandomNumber  Minimum=M_cmin  Maximum=M_cmax  SampleTime=1
  x_l : Outport
  y_l : Outport  Port=2
  v_xl : Outport  Port=3
  v_yl : Outport  Port=4
  m_l (sim) : Outport  Port=5
  wires:
  Sum/1 -> Divide/1
  Divide/1 -> Integrator3/1
  theta_l/1 -> Cos/1, Sin/1
  F_hw/1 -> Gain1/1
  Gain1/1 -> Product/1, Product1/1
  Sin/1 -> Product/2
  Product/1 -> Sum/1
  Switch1/1 -> F_cx/1(h_c), F_cy/3(h_c)
  Product1/1 -> Sum1/1
  Cos/1 -> Product1/2
  F_cy/1(F_cy) -> Sum1/2, Scope/1  "F_cy"
  Divide1/1 -> Integrator2/1
  Sum1/1 -> Divide1/1
  Integrator/1 -> x_l/1  "x_l"
  Integrator3/1 -> v_xl/1, F_cx/4(v_lx), Integrator/1
  Integrator2/1 -> v_yl/1, F_cy/2(v_ly), Integrator1/1
  Integrator1/1 -> y_l/1, F_cx/3(y_l), F_cy/1(y_l)  "y_l"
  y_c0/1 -> F_cx/2(y_c0), F_cy/4(y_c0)
  F_cx/1(F_cx) -> Sum/2  "F_cx"
  TLK/1 -> Sample and Hold/Trigger, Switch/2  "TLK"
  Switch/1 -> Sum2/2  "M_c"
  Constant3/1 -> Sum2/1
  Sum2/1 -> Gain/1, Divide1/2, Divide/2, m_l (sim)/1  "m_l"
  Uniform Random Number/1 -> Sample and Hold/1
  Sample and Hold/1 -> Switch/1
  Constant/1 -> Switch/3
  Constant1/1 -> Switch1/1
  Constant2/1 -> Switch1/3
  Gain/1 -> Sum1/3
  spreader_has_load/1 -> Switch1/2

== system modelo_f_HIL_ST/Nivel 2/Subsistema físico/Carro ==
  F_tw : Inport
  F_hw : Inport  Port=2
  theta_l : Inport  Port=3
  Gain : Gain  Gain=2
  Gain1 : Gain  Gain=b_t
  Gain2 : Gain  Gain=1/M_t
  Integrator : Integrator  InitialCondition=v_t0
  Integrator1 : Integrator  InitialCondition=x_t0
  Product : Product
  Sin : Trigonometry
  Sum : Sum  Inputs=-++
  x_t : Outport
  v_t : Outport  Port=2
  a_t : Outport  Port=3
  wires:
  F_tw/1 -> Sum/3
  F_hw/1 -> Gain/1
  Gain/1 -> Product/1
  theta_l/1 -> Sin/1
  Sin/1 -> Product/2
  Product/1 -> Sum/2
  Integrator/1 -> v_t/1, Integrator1/1, Gain1/1  "v_t"
  Sum/1 -> Gain2/1
  Gain2/1 -> a_t/1, Integrator/1  "dv_t/dt"
  Integrator1/1 -> x_t/1
  Gain1/1 -> Sum/1

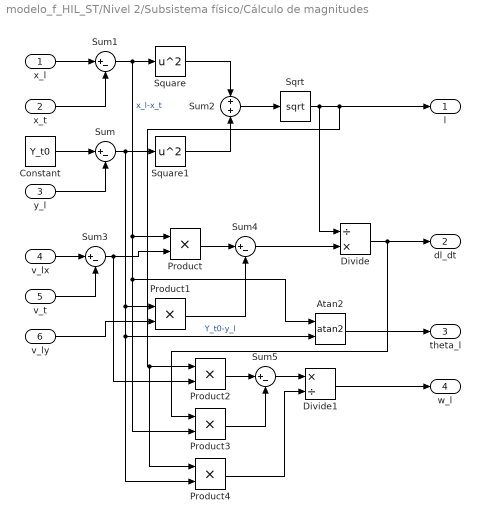
== system modelo_f_HIL_ST/Nivel 2/Subsistema físico/Cálculo de magnitudes ==
  x_l : Inport
  x_t : Inport  Port=2
  y_l : Inport  Port=3
  v_lx : Inport  Port=4
  v_t : Inport  Port=5
  v_ly : Inport  Port=6
  Atan2 : Trigonometry  Operator=atan2
  Constant : Constant  Value=Y_t0
  Divide : Product  Inputs=/*
  Divide1 : Product  Inputs=*/
  Product{,1..4} (5 alike) : Product
  Sqrt : Sqrt
  Square : Math  Operator=square
  Square1 : Math  Operator=square
  Sum{,1,3..5} (5 alike) : Sum  Inputs=|+-
  Sum2 : Sum  Inputs=+|+
  l : Outport
  dl_dt : Outport  Port=2
  theta_l : Outport  Port=3
  w_l : Outport  Port=4
  wires:
  Constant/1 -> Sum/1
  y_l/1 -> Sum/2
  x_l/1 -> Sum1/1
  x_t/1 -> Sum1/2
  Sum1/1 -> Product3/2, Atan2/1, Product/1, Square/1  "x_l-x_t"
  Sum/1 -> Product4/2, Atan2/2, Product1/1, Square1/1  "Y_t0-y_l"
  Square/1 -> Sum2/1
  Square1/1 -> Sum2/2
  Sum2/1 -> Sqrt/1
  Sqrt/1 -> Divide/1, Product4/1, Product2/1, l/1
  v_lx/1 -> Sum3/1
  v_t/1 -> Sum3/2
  Sum3/1 -> Product2/2, Product/2
  Product/1 -> Sum4/1
  v_ly/1 -> Product1/2
  Product1/1 -> Sum4/2
  Sum4/1 -> Divide/2
  Divide/1 -> Product3/1, dl_dt/1
  Atan2/1 -> theta_l/1
  Divide1/1 -> w_l/1
  Product2/1 -> Sum5/1
  Product3/1 -> Sum5/2
  Sum5/1 -> Divide1/1
  Product4/1 -> Divide1/2

== system modelo_f_HIL_ST/Nivel 2/Subsistema físico/Field Weaking Izaje ==
  w_hm : Inport
  Abs : Abs  SaturateOnIntegerOverflow=off
  Constant : Constant  Value=w_hm_rated
  Divide : Product  Inputs=*/
  Gain : Gain  Gain=T_hmMax
  Max : MinMax  Function=max  Inputs=2
  Square : Math  Operator=square
  T_hm_max : Outport
  wires:
  w_hm/1 -> Abs/1
  Constant/1 -> Divide/1, Max/2
  Divide/1 -> Square/1
  Square/1 -> Gain/1
  Gain/1 -> T_hm_max/1
  Abs/1 -> Max/1
  Max/1 -> Divide/2

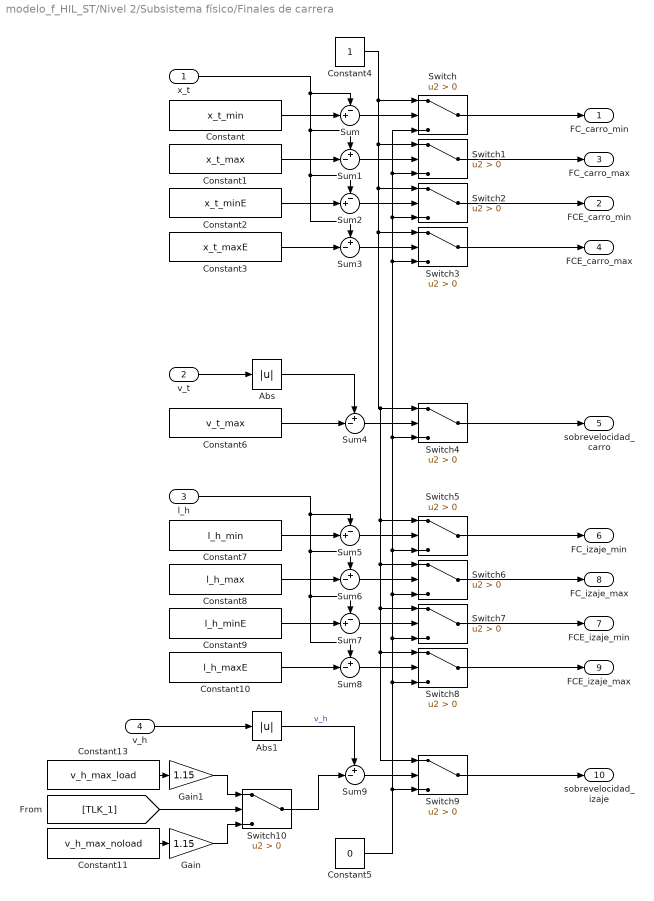
== system modelo_f_HIL_ST/Nivel 2/Subsistema físico/Finales de carrera ==
  x_t : Inport
  v_t : Inport  Port=2
  l_h : Inport  Port=3
  v_h : Inport  Port=4
  Abs : Abs  SaturateOnIntegerOverflow=off
  Abs1 : Abs  SaturateOnIntegerOverflow=off
  Constant : Constant  Value=x_t_min
  Constant1 : Constant  Value=x_t_max
  Constant10 : Constant  Value=l_h_maxE
  Constant11 : Constant  Value=v_h_max_noload
  Constant13 : Constant  Value=v_h_max_load
  Constant2 : Constant  Value=x_t_minE
  Constant3 : Constant  Value=x_t_maxE
  Constant4 : Constant
  Constant5 : Constant  Value=0
  Constant6 : Constant  Value=v_t_max
  Constant7 : Constant  Value=l_h_min
  Constant8 : Constant  Value=l_h_max
  Constant9 : Constant  Value=l_h_minE
  Gain : Gain  Gain=1.15
  Gain1 : Gain  Gain=1.15
  Sum{,2,5,7} (4 alike) : Sum  Inputs=-+|
  Sum{1,3..4,6,8..9} (6 alike) : Sum  Inputs=+-|
  Switch{,1..10} (11 alike) : Switch  Criteria=u2 > Threshold  SaturateOnIntegerOverflow=off  InputSameDT=off
  FC_carro_min : Outport
  FCE_carro_min : Outport  Port=2
  FC_carro_max : Outport  Port=3
  FCE_carro_max : Outport  Port=4
  sobrevelocidad_carro : Outport  Port=5
  FC_izaje_min : Outport  Port=6
  FCE_izaje_min : Outport  Port=7
  FC_izaje_max : Outport  Port=8
  FCE_izaje_max : Outport  Port=9
  sobrevelocidad_izaje : Outport  Port=10
  wires:
  Constant/1 -> Sum/2
  Constant1/1 -> Sum1/2
  Constant2/1 -> Sum2/2
  Constant3/1 -> Sum3/2
  x_t/1 -> Sum/1, Sum1/1, Sum2/1, Sum3/1
  Sum/1 -> Switch/2
  Constant4/1 -> Switch2/1, Switch9/1, Switch8/1, Switch7/1, Switch6/1, Switch5/1, Switch4/1, Switch3/1, Switch1/1, Switch/1
  Sum1/1 -> Switch1/2
  Sum2/1 -> Switch2/2
  Sum3/1 -> Switch3/2
  Switch/1 -> FC_carro_min/1
  Switch1/1 -> FC_carro_max/1
  Switch2/1 -> FCE_carro_min/1
  Switch3/1 -> FCE_carro_max/1
  v_t/1 -> Abs/1
  Constant6/1 -> Sum4/2
  Sum4/1 -> Switch4/2
  Abs/1 -> Sum4/1
  Switch4/1 -> sobrevelocidad_carro/1
  Switch7/1 -> FCE_izaje_min/1
  Switch6/1 -> FC_izaje_max/1
  l_h/1 -> Sum5/1, Sum6/1, Sum7/1, Sum8/1
  Sum7/1 -> Switch7/2
  Switch5/1 -> FC_izaje_min/1
  Constant7/1 -> Sum5/2
  Constant10/1 -> Sum8/2
  Constant9/1 -> Sum7/2
  Sum6/1 -> Switch6/2
  Constant8/1 -> Sum6/2
  Sum8/1 -> Switch8/2
  Constant5/1 -> Switch9/3, Switch8/3, Switch6/3, Switch5/3, Switch1/3, Switch/3, Switch2/3, Switch3/3, Switch4/3, Switch7/3
  Switch8/1 -> FCE_izaje_max/1
  Sum5/1 -> Switch5/2
  Constant11/1 -> Gain/1
  v_h/1 -> Abs1/1
  Abs1/1 -> Sum9/1  "v_h"
  Sum9/1 -> Switch9/2
  Switch9/1 -> sobrevelocidad_izaje/1
  Gain/1 -> Switch10/3
  [TLK_1] -> Switch10/2
  Switch10/1 -> Sum9/2
  Constant13/1 -> Gain1/1
  Gain1/1 -> Switch10/1

== system modelo_f_HIL_ST/Nivel 2/Subsistema físico/Moduladores de torque ==
  T_tm* : Inport
  T_hm* : Inport  Port=2
  T_hmMax : Inport  Port=3
  +-T_tmMax : Saturate  UpperLimit=+T_tmMax  LowerLimit=-T_tmMax
  Gain : Gain  Gain=1/tau_tm
  Gain1 : Gain  Gain=1/tau_tm
  Gain2 : Gain  Gain=-1
  Integrator : Integrator
  Integrator1 : Integrator
  Saturation Dynamic : simulink/Discontinuities/Saturation Dynamic  OutMin=[]  OutMax=[]  OutDataTypeStr=Inherit: Same as second input  OutDataType=fixdt(1, 16)  OutScaling=2^-10  DoSatur=off
  Sum : Sum  Inputs=|+-
  Sum1 : Sum  Inputs=|+-
  T_tm : Outport
  T_hm : Outport  Port=2
  wires:
  +-T_tmMax/1 -> T_tm/1
  Gain/1 -> Integrator/1
  Integrator/1 -> Sum/2, +-T_tmMax/1
  T_tm*/1 -> Sum/1
  Sum/1 -> Gain/1
  Gain1/1 -> Integrator1/1
  Sum1/1 -> Gain1/1
  Integrator1/1 -> Sum1/2, Saturation Dynamic/2
  T_hm*/1 -> Sum1/1
  Saturation Dynamic/1 -> T_hm/1
  T_hmMax/1 -> Gain2/1, Saturation Dynamic/1
  Gain2/1 -> Saturation Dynamic/3

== system modelo_f_HIL_ST/Nivel 2/Subsistema físico/Accionamiento Carro/Subsystem ==
  BRK_t : Inport
  w_tm : Inport  Port=2
  Constant : Constant  Value=0
  Gain : Gain  Gain=b_tb
  Gain1 : Gain  Gain=-T_tbMax
  Switch : Switch  Criteria=u2 ~= 0  SaturateOnIntegerOverflow=off  InputSameDT=off
  Tanh : Trigonometry  Operator=tanh
  T_tb : Outport
  wires:
  BRK_t/1 -> Switch/2
  Constant/1 -> Switch/1
  Gain/1 -> Tanh/1
  w_tm/1 -> Gain/1
  Switch/1 -> T_tb/1
  Tanh/1 -> Gain1/1
  Gain1/1 -> Switch/3

== system modelo_f_HIL_ST/Nivel 2/Subsistema físico/Accionamiento Izaje/Freno de operación ==
  BRK_h : Inport
  w_hm : Inport  Port=2
  Constant : Constant  Value=0
  Gain : Gain  Gain=b_hb
  Gain1 : Gain  Gain=-T_hbMax
  Switch : Switch  Criteria=u2 ~= 0  SaturateOnIntegerOverflow=off  InputSameDT=off
  Tanh : Trigonometry  Operator=tanh
  T_hb : Outport
  wires:
  BRK_h/1 -> Switch/2
  Constant/1 -> Switch/1
  Gain/1 -> Tanh/1
  w_hm/1 -> Gain/1
  Switch/1 -> T_hb/1
  Tanh/1 -> Gain1/1
  Gain1/1 -> Switch/3

== system modelo_f_HIL_ST/Nivel 2/Subsistema físico/Accionamiento Izaje/Freno de operación1 ==
  BRK_hE : Inport
  w_hd : Inport  Port=2
  Constant : Constant  Value=0
  Gain : Gain  Gain=b_hd
  Gain1 : Gain  Gain=-T_hEbMax
  Switch : Switch  Criteria=u2 ~= 0  SaturateOnIntegerOverflow=off  InputSameDT=off
  Tanh : Trigonometry  Operator=tanh
  T_hEb : Outport
  wires:
  BRK_hE/1 -> Switch/2
  Constant/1 -> Switch/1
  Gain/1 -> Tanh/1
  w_hd/1 -> Gain/1
  Switch/1 -> T_hEb/1
  Tanh/1 -> Gain1/1
  Gain1/1 -> Switch/3

== system modelo_f_HIL_ST/Nivel 2/Subsistema físico/Cable izaje/Calculo K_hw ==
  l_h : Inport
  Constant : Constant  Value=110
  Constant1 : Constant  Value=k_wu
  Divide : Product  Inputs=*/
  Gain : Gain  Gain=2
  Sum : Sum  Inputs=|++
  K_hw : Outport
  wires:
  l_h/1 -> Gain/1
  Gain/1 -> Sum/1
  Constant/1 -> Sum/2
  Sum/1 -> Divide/2
  Constant1/1 -> Divide/1
  Divide/1 -> K_hw/1

== system modelo_f_HIL_ST/Nivel 2/Subsistema físico/Cable izaje/Calculo b_hw ==
  l_h : Inport
  Constant : Constant  Value=110
  Gain : Gain  Gain=2
  Gain1 : Gain  Gain=b_wu
  Sum : Sum  Inputs=|++
  b_hw : Outport
  wires:
  l_h/1 -> Gain/1
  Gain/1 -> Sum/1
  Constant/1 -> Sum/2
  Sum/1 -> Gain1/1
  Gain1/1 -> b_hw/1

== system modelo_f_HIL_ST/Nivel 2/Subsistema físico/Carga/F_cx ==
  h_c : Inport
  y_c0 : Inport  Port=2
  y_l : Inport  Port=3
  v_lx : Inport  Port=4
  Constant : Constant  Value=0
  Gain : Gain  Gain=-b_cx
  Sum : Sum  Inputs=|+-
  Sum1 : Sum  Inputs=|-+
  Switch : Switch  Criteria=u2 > Threshold  SaturateOnIntegerOverflow=off  InputSameDT=off
  F_cx : Outport
  wires:
  y_l/1 -> Sum/1
  h_c/1 -> Sum/2
  Sum/1 -> Sum1/1
  y_c0/1 -> Sum1/2
  Sum1/1 -> Switch/2
  Constant/1 -> Switch/3
  v_lx/1 -> Gain/1
  Gain/1 -> Switch/1
  Switch/1 -> F_cx/1

== system modelo_f_HIL_ST/Nivel 2/Subsistema físico/Carga/F_cy ==
  y_l : Inport
  v_ly : Inport  Port=2
  h_c : Inport  Port=3
  y_c0 : Inport  Port=4
  Constant1 : Constant  Value=0
  Gain : Gain  Gain=K_cy
  Gain1 : Gain  Gain=b_cy
  Sum : Sum  Inputs=|+-
  Sum1 : Sum  Inputs=|-+
  Sum2 : Sum  Inputs=|+-
  Sum3 : Sum  Inputs=|-+
  switch : Switch  Criteria=u2 > Threshold  SaturateOnIntegerOverflow=off  InputSameDT=off
  F_cy : Outport
  wires:
  switch/1 -> F_cy/1
  Sum2/1 -> switch/1
  Constant1/1 -> switch/3
  Sum/1 -> Sum3/1, Sum1/1
  y_l/1 -> Sum/1
  h_c/1 -> Sum/2
  y_c0/1 -> Sum3/2, Sum1/2
  Sum1/1 -> Gain/1
  Gain/1 -> Sum2/1
  v_ly/1 -> Gain1/1
  Gain1/1 -> Sum2/2
  Sum3/1 -> switch/2

== matlab function modelo_f_HIL_ST/Nivel 2/MATLAB Function4 ==
  data: T_hm input; out_wm_hm_hat output; F_hw input; theta_hm input; out_theta_hm_hat output
function [out_wm_hm_hat, out_theta_hm_hat] = fcn(T_hm, F_hw, theta_hm)
    persistent Lh1 Lh2 T_s b_hEq J_hEq r_hd i_h ...
               w_hat_prev dw_hat_prev theta_hat e_theta_prev

    if isempty(Lh1)
        Lh1 = 9.5197;
        Lh2 = 20.3903;
        J_hEq = 37.8512;
        b_hEq = 18.0165;
        r_hd  = 0.75;
        i_h   = 22;
        T_s   = 0.001;

        w_hat_prev   = 0;
        dw_hat_prev  = 0;
        theta_hat    = theta_hm;
        e_theta_prev = 0;
    end

    % Error de posicion actual
    e_theta = theta_hm - theta_hat;

    % Derivada de velocidad: solo modelo + L2 (estado de velocidad "limpio")
    dw_hat = (1/J_hEq) * (T_hm - w_hat_prev*b_hEq - F_hw*(r_hd/i_h)) + Lh2*e_theta;

    % Integracion trapezoidal de velocidad
    w_hat = w_hat_prev + T_s * (dw_hat_prev + dw_hat) / 2;

    % Derivada de posicion: velocidad + L1 (correccion SOLO aca)
    dtheta_hat      = w_hat      + Lh1 * e_theta;
    dtheta_hat_prev = w_hat_prev + Lh1 * e_theta_prev;

    % Integracion trapezoidal de posicion
    theta_hat = theta_hat + T_s * (dtheta_hat_prev + dtheta_hat) / 2;

    % Actualizar memorias
    w_hat_prev   = w_hat;
    dw_hat_prev  = dw_hat;
    e_theta_prev = e_theta;

    out_wm_hm_hat    = w_hat;
    out_theta_hm_hat = theta_hat;
end
